simulink model "outter_tanks_init"  (R2020a)
settings: Solver=FixedStepAuto  StartTime=0.0  StopTime=inf  FixedStep=1  RelTol=1e-3
libraries: modbusMatLib x12, simulink x4, realtime_pacer_lib x1
(part 2 of 2)

== matlab function outter_tanks_init/MATLAB Function ==
  data: ex_tank1 input; initialized output; ex_tank2 input
function initialized = Termination(ex_tank1, ex_tank2)
    if ex_tank1<150 && ex_tank2 < 150
        initialized = 1;
    else
        initialized = 0;
    end
end

== matlab function outter_tanks_init/MATLAB Function1 ==
  settings: updateMethod=DISCRETE
  data: ex_tank1 input; pump1_setting output
function pump1_setting = empty_outter_tank(ex_tank1)
    if ex_tank1<150                      
        pump1_setting=0;
    else
        pump1_setting = 8;
    end
end

== matlab function outter_tanks_init/MATLAB Function3 ==
  data: ex_tank_2 input; pump2_setting output
function pump2_setting = empty_outter_tank(ex_tank_2)
    if ex_tank_2 < 150
        pump2_setting = 0;
    else
        pump2_setting = 14;
end

== matlab function outter_tanks_init/MATLAB Function4 ==
  data: buffer_tank_level input; open_buffer_tank output; disturbance_tank_level input; old_output input
function open_buffer_tank = buffers_control(buffer_tank_level, disturbance_tank_level, old_output)

if buffer_tank_level > 600
    open_buffer_tank = 0;
elseif disturbance_tank_level > 600
    open_buffer_tank = 1;
elseif buffer_tank_level < 250
    open_buffer_tank = 1;
elseif disturbance_tank_level < 250
    open_buffer_tank = 0;
else
    open_buffer_tank = old_output;
end
end

== matlab function outter_tanks_init/Buffers water distribution/MATLAB Function4 ==
  data: buffer_tank_level input; tank_select output; disturbance_tank_level input; old_output input
function tank_select = buffers_control(buffer_tank_level, disturbance_tank_level, old_output)

    if 300 > buffer_tank_level
        tank_select = 1;
    elseif 300 > disturbance_tank_level
        tank_select = 0;
    else
        tank_select = old_output;
    end
end
